simulink model "Trim_Model"  (R2014b)
settings: Solver=ode23tb  StartTime=0.0  StopTime=inf  FixedStep=0.001  MaxStep=0.01  RelTol=1e-5
values from neighbouring files (symbols this model uses):
  A_x = 0.015    [SetupComplete.m]
  A_y = A_x    (= 0.015)    [SetupComplete.m]
  A_z = 0.16    [SetupComplete.m]
  C_x = 1.2    [SetupComplete.m]
  C_y = C_x    (= 1.2)    [SetupComplete.m]
  C_z = 2.2    [SetupComplete.m]
  CG_0 = [0,0,0.02]'    [SetupComplete.m]
  h = 0.08    [SetupComplete.m]
  h_M = 0.064    [SetupComplete.m]
  I_BAC_0 = [ Ix,0,Ixz;0,Iy,0;Ixz,0,Iz]    [SetupComplete.m]
  l = 0.345    [SetupComplete.m]
  l_arm = 0.264    [SetupComplete.m]
  m = 3.51    [SetupComplete.m]
  m_0 = 2.61    [SetupComplete.m]
  m_M = 0.300    (= 0.3)    [SetupComplete.m]
  rho = 1.15    [SetupComplete.m]
  Rotation_sign = [ 1,-1,-1]    [SetupComplete.m]
undefined symbols (not defined in the file or in its folder): Throttle_Hover
libraries: simulink_extras x5, XXCopter_C x3, dspmtrx3 x2, aerolibtransform2 x1
settings Model: ExtModeTrigDuration=5000  Creator=DavidTorres  LastModifiedBy=david.torres
settings SolverCC: SolverResetMethod=Robust  PositivePriorityOrder=on
settings DataIOCC: ExternalInput=getinputstruct(op_trim1)  InitialState=getstatestruct(op_trim1)  SignalLoggingSaveFormat=ModelDataLogs  Refine=10
settings OptimizationCC: InlineParams=on  ExpressionDepthLimit=2147483647
settings DebuggingCC: UnderspecifiedInitializationDetection=Classic  MergeDetectMultiDrivingBlocksExec=none  FcnCallInpInsideContextMsg=UseLocalSettings  StateNameClashWarn=warning
settings RTWCC: SystemTargetFile=quarc_windows.tlc  TemplateMakefile=quarc_default_tmf  Description=QUARC Win32 Target  ProcessScript=quarc_windows_make_rtw_hook
settings STFCustomTargetCC: TargetPreCompLibLocation=C:\PROGRA~2\QUARC\lib\2011a\windows\release  CodeReplacementLibrary=C89/C90 (ANSI)  GeneratePreprocessorConditionals=Disable all  CPPClassGenCompliant=on  SystemTargetFile=quarc_windows.tlc
settings GRTTargetCC: TargetPreCompLibLocation=C:\PROGRA~2\QUARC\lib\2011a\windows\release  CodeReplacementLibrary=C89/C90 (ANSI)  ParMdlRefBuildCompliant=off  CompOptLevelCompliant=off  ConcurrentExecutionCompliant=off  CombineOutputUpdateFcns=off  MatFileLogging=off  GRTInterface=on  ExtMode=on  ExtModeMexFile=quarc_comm

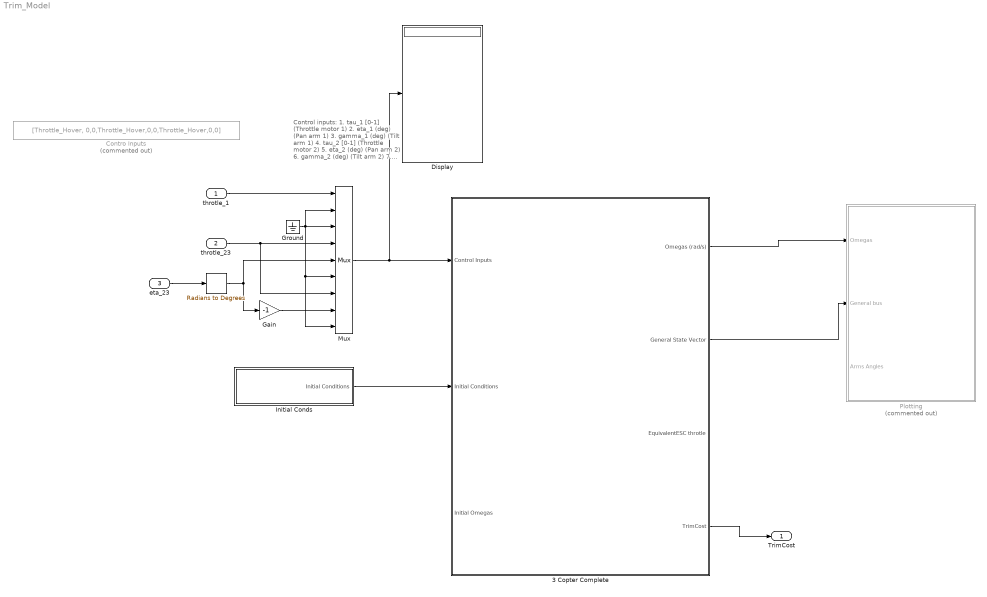
== system Trim_Model ==
  note: Control inputs:
      | 1. tau_1 [0-1] (Throttle motor 1)
      | 2. eta_1 (deg)  (Pan arm 1)
      | 3. gamma_1 (deg)  (Tilt arm 1)
      |
      | 4. tau_2 [0-1] (Throttle motor 2)
      | 5. eta_2 (deg)  (Pan arm 2)
      | 6. gamma_2 (deg)  (Tilt arm 2)
      |
      | 7. tau_3 [0-1] (Throttle motor 3)
      | 8. eta_3 (deg)  (Pan arm  3)
      | 9. gamma_3 (deg)  (Tilt arm 3)
  throtle_1 : Inport
  throtle_23 : Inport  Port=2
  eta_23 : Inport  Port=3
  " " : simulink_extras/Transformations/Radians to Degrees
  3 Copter Complete : Subsystem  TreatAsAtomicUnit=on
  Contro Inputs : Constant  Commented=on  Value=[Throttle_Hover, 0,0,Throttle_Hover,0,0,Throttle_Hover,0,0]
  Display : Display
  Gain : Gain  Gain=-1
  Ground : Ground
  Initial Conds : Subsystem  TreatAsAtomicUnit=on
  Mux : Mux  Inputs=9
  Plotting : Subsystem  Commented=on
  TrimCost : Outport
  wires:
  Initial Conds/1(Initial Conditions) -> 3 Copter Complete/2(Initial Conditions)
  Mux/1 -> Display/1, 3 Copter Complete/1(Control Inputs)
  3 Copter Complete/2(General State Vector) -> Plotting/2(General bus)
  3 Copter Complete/1(Omegas (rad/s)) -> Plotting/1(Omegas)
  ? -> Plotting/3(Arms Angles)
  3 Copter Complete/4(TrimCost) -> TrimCost/1
  throtle_1/1 -> Mux/1
  throtle_23/1 -> Mux/7, Mux/4
  Ground/1 -> Mux/2, Mux/6, Mux/9, Mux/3
  eta_23/1 -> " "/1
  " "/1 -> Gain/1, Mux/5
  Gain/1 -> Mux/8

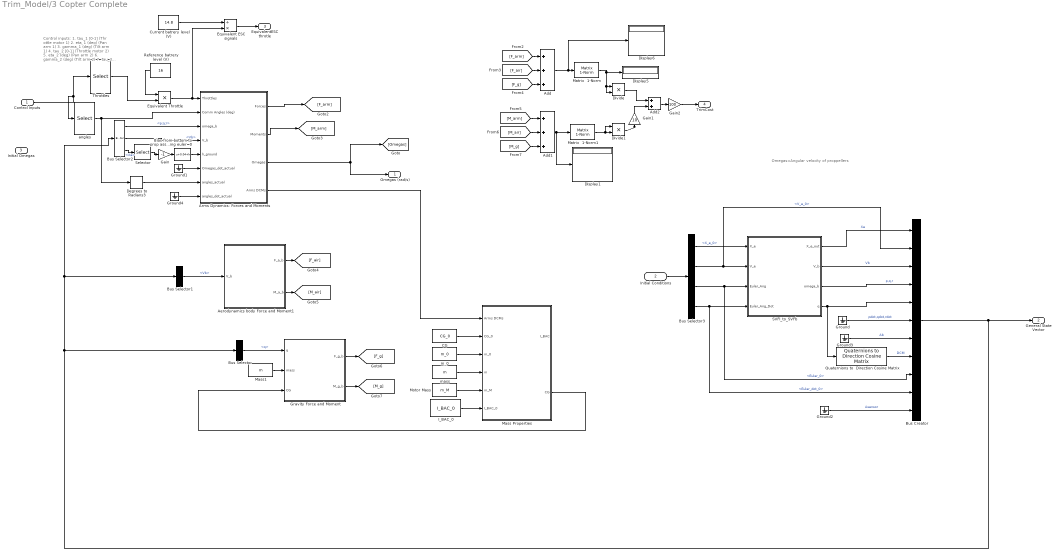
== system Trim_Model/3 Copter Complete ==
  note: Omegas=Angular velocity of proppellers
  note: Control inputs:
      | 1. tau_1 [0-1] (Thr ottle motor 1)
      | 2. eta_1 (deg)  (Pan arm 1)
      | 3. gamma_1 (deg)  (Tilt arm 1)
      |
      | 4. tau_2 [0-1] (Throttle motor 2)
      | 5. eta_2 (deg)  (Pan arm 2)
      | 6. gamma_2 (deg)  (Tilt arm 2)
      |
      | 7. tau_3 [0-1] (Throttle motor 3)
      | 8. eta_3 (deg)  (Pan arm  3)
      | 9. gamma_3 (deg)  (Tilt arm 3)
  Control Inputs : Inport
  Initial Conditions : Inport  Port=2
  Initial Omegas : Inport  Port=3
  Add : Sum  Inputs=+++
  Add1 : Sum  Inputs=+++
  Add2 : Sum
  Aerodynamics body Force and Moment1 : MATLAB Function  TreatAsAtomicUnit=on
  Arms Dynamics: Forces and Moments : Subsystem
  Bias from bottom to prop assuming euler=0 : Bias  Bias=0.04+h
  Bus Creator : BusCreator  Inputs=11
  Bus Selector : BusSelector  OutputSignals=q
  Bus Selector1 : BusSelector  OutputSignals=Vb
  Bus Selector2 : BusSelector  OutputSignals=p;q;r,Vb,Xe
  Bus Selector3 : BusSelector  OutputSignals=X_e_0,V_e_0,Euler_0,Euler_dot_0
  CG : Constant  Value=CG_0
  Current batrery level (V) : Constant  Value=14.8
  Degrees to Radians3 : simulink_extras/Transformations/Degrees to Radians
  Display1 : Display
  Display5 : Display
  Display6 : Display
  Divide : Product  Inputs=**
  Divide1 : Product  Inputs=**
  Equivalent ESC signals : Product  Inputs=/*
  Equivalent Throttle : Product  Inputs=**
  Gain : Gain  Gain=-1
  Gain1 : Gain  Gain=10
  Gain2 : Gain  Gain=100
  Gravity Force and Moment : MATLAB Function  TreatAsAtomicUnit=on
  Ground{,1..4} (5 alike) : Ground
  I_BAC_0 : Constant  Value=I_BAC_0
  Mass Properties : Subsystem  TreatAsAtomicUnit=on
  Mass1 : Constant  Value=m
  Matrix  1-Norm : dspmtrx3/Matrix  1-Norm  outputDataTypeStr=Inherit: Same as accumulator  outputLastDataTypeStr=Inherit: Same as accumulator  outputMin=[]  outputMax=[]  roundingMode=Floor  overflowMode=off
  Matrix  1-Norm1 : dspmtrx3/Matrix  1-Norm  outputDataTypeStr=Inherit: Same as accumulator  outputLastDataTypeStr=Inherit: Same as accumulator  outputMin=[]  outputMax=[]  roundingMode=Floor  overflowMode=off
  Motor Mass : Constant  Value=m_M
  Quaternions to  Direction Cosine Matrix : aerolibtransform2/Quaternions to  Direction Cosine Matrix
  Reference batrery level (V) : Constant  Value=16
  SVFI_to_SVFb : MATLAB Function  TreatAsAtomicUnit=on
  Selector : Selector  InputPortWidth=3  Indices=3
  Throttles : Selector  InputPortWidth=9  Indices=[1,4,7]
  "angles " : Selector  InputPortWidth=9  Indices=[2,3,5,6,8,9]
  m_0 : Constant  Value=m_0
  mass : Constant  Value=m
  Omegas (rad/s) : Outport
  General State Vector : Outport  Port=2
  EquivalentESC throtle : Outport  Port=3
  TrimCost : Outport  Port=4
  wires:
  SVFI_to_SVFb/3(omega_b) -> Bus Creator/4  "p,q,r"
  SVFI_to_SVFb/2(V_b) -> Bus Creator/3  "Vb"
  SVFI_to_SVFb/4(q) -> Quaternions to  Direction Cosine Matrix/1, Bus Creator/5
  Ground/1 -> Bus Creator/6  "pdot,qdot,rdot"
  SVFI_to_SVFb/1(X_e_out) -> Bus Creator/1  "Xe"
  Ground3/1 -> Bus Creator/7  "Ab"
  Bus Selector/1 -> Gravity Force and Moment/1(q)  "<q>"
  Bus Selector1/1 -> Aerodynamics body Force and Moment1/1(V_b)  "<Vb>"
  Bus Selector2/1 -> Arms Dynamics: Forces and Moments/3(omega_b)  "<p;q;r>"
  Bus Selector2/2 -> Arms Dynamics: Forces and Moments/4(V_b)  "<Vb>"
  Mass1/1 -> Gravity Force and Moment/2(mass)
  Mass Properties/2(CG) -> Gravity Force and Moment/3(CG)
  Bus Selector2/3 -> Selector/1  "<Xe>"
  Selector/1 -> Gain/1
  Arms Dynamics: Forces and Moments/1(Forces) -> [F_arm]
  Arms Dynamics: Forces and Moments/2(Moments) -> [M_arm]
  Aerodynamics body Force and Moment1/1(F_a_b) -> [F_air]
  Aerodynamics body Force and Moment1/2(M_a_b) -> [M_air]
  Gravity Force and Moment/1(F_g_b) -> [F_g]
  Gravity Force and Moment/2(M_g_b) -> [M_g]
  [F_arm] -> Add/1
  [F_air] -> Add/2
  [F_g] -> Add/3
  [M_arm] -> Add1/1
  [M_g] -> Add1/3
  [M_air] -> Add1/2
  Ground2/1 -> Bus Creator/11  "Asensor"
  Throttles/1 -> Equivalent Throttle/2
  Control Inputs/1 -> "angles "/1, Throttles/1
  "angles "/1 -> Arms Dynamics: Forces and Moments/2(Comm Angles (deg)), Degrees to Radians3/1
  Arms Dynamics: Forces and Moments/4(Arms DCMs) -> Mass Properties/1(Arms DCMs)
  CG/1 -> Mass Properties/2(CG_0)
  Motor Mass/1 -> Mass Properties/5(m_M)
  I_BAC_0/1 -> Mass Properties/6(I_BAC_0)
  m_0/1 -> Mass Properties/3(m_0)
  mass/1 -> Mass Properties/4(m)
  Arms Dynamics: Forces and Moments/3(Omegas) -> [Omegas], Omegas (rad/s)/1
  Bus Creator/1 -> Bus Selector2/1, Bus Selector1/1, Bus Selector/1, General State Vector/1
  Equivalent Throttle/1 -> Arms Dynamics: Forces and Moments/1(Throttles), Equivalent ESC signals/2
  Reference batrery level (V)/1 -> Equivalent Throttle/1
  Current batrery level (V)/1 -> Equivalent ESC signals/1
  Equivalent ESC signals/1 -> EquivalentESC throtle/1
  Initial Conditions/1 -> Bus Selector3/1
  Bus Selector3/1 -> SVFI_to_SVFb/1(X_e)  "<X_e_0>"
  Bus Selector3/2 -> Bus Creator/2, SVFI_to_SVFb/2(V_e)  "<V_e_0>"
  Bus Selector3/3 -> Bus Creator/9, SVFI_to_SVFb/3(Euler_Ang)  "<Euler_0>"
  Bus Selector3/4 -> Bus Creator/10, SVFI_to_SVFb/4(Euler_Ang_Dot)  "<Euler_dot_0>"
  Quaternions to  Direction Cosine Matrix/1 -> Bus Creator/8  "DCM"
  Add/1 -> Display6/1, Matrix  1-Norm/1
  Add1/1 -> Display1/1, Matrix  1-Norm1/1
  Add2/1 -> Gain2/1
  Gain1/1 -> Add2/2
  Matrix  1-Norm1/1 -> Divide1/1, Divide1/2
  Matrix  1-Norm/1 -> Divide/2, Divide/1, Display5/1
  Gain2/1 -> TrimCost/1
  Divide/1 -> Add2/1
  Divide1/1 -> Gain1/1
  Degrees to Radians3/1 -> Arms Dynamics: Forces and Moments/7(angles_actual)
  Ground1/1 -> Arms Dynamics: Forces and Moments/6(Omegas_dot_actual)
  Ground4/1 -> Arms Dynamics: Forces and Moments/8(angles_dot_actual)
  Gain/1 -> Bias from bottom to prop assuming euler=0/1
  Bias from bottom to prop assuming euler=0/1 -> Arms Dynamics: Forces and Moments/5(h_ground)

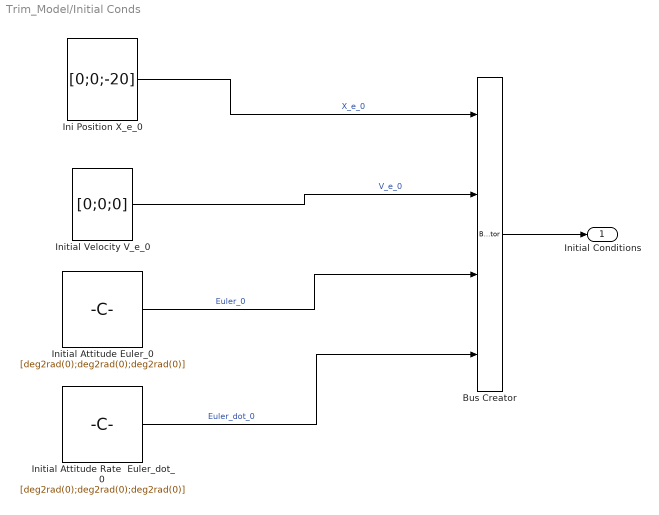
== system Trim_Model/Initial Conds ==
  Bus Creator : BusCreator
  Ini Position X_e_0 : Constant  Value=[0;0;-20]
  Initial Attitude Euler_0 : Constant  Value=[deg2rad(0);deg2rad(0);deg2rad(0)]
  Initial Attitude Rate  Euler_dot_0 : Constant  Value=[deg2rad(0);deg2rad(0);deg2rad(0)]
  Initial Velocity V_e_0 : Constant  Value=[0;0;0]
  Initial Conditions : Outport
  wires:
  Ini Position X_e_0/1 -> Bus Creator/1  "X_e_0"
  Initial Velocity V_e_0/1 -> Bus Creator/2  "V_e_0"
  Initial Attitude Euler_0/1 -> Bus Creator/3  "Euler_0"
  Initial Attitude Rate  Euler_dot_0/1 -> Bus Creator/4  "Euler_dot_0"
  Bus Creator/1 -> Initial Conditions/1

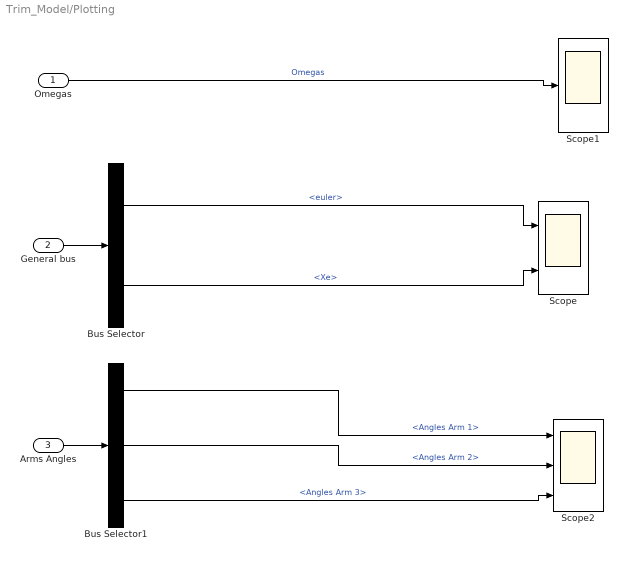
== system Trim_Model/Plotting ==
  Omegas : Inport
  General bus : Inport  Port=2
  Arms Angles : Inport  Port=3
  Bus Selector : BusSelector  OutputSignals=euler,Xe
  Bus Selector1 : BusSelector  OutputSignals=Angles Arm 1,Angles Arm 2,Angles Arm 3
  Scope : Scope  NumInputPorts=2
      settings: YMin=-3.5~-110  YMax=3.5~40
  Scope1 : Scope
      settings: TimeRange=5  YMin=0  YMax=700
  Scope2 : Scope  NumInputPorts=3
      settings: ShowLegends=on  YMin=-5~-5~-5  YMax=5~5~5  SaveName=ScopeData2
  wires:
  General bus/1 -> Bus Selector/1
  Bus Selector/1 -> Scope/1  "<euler>"
  Omegas/1 -> Scope1/1  "Omegas"
  Arms Angles/1 -> Bus Selector1/1
  Bus Selector1/3 -> Scope2/3  "<Angles Arm 3>"
  Bus Selector1/2 -> Scope2/2  "<Angles Arm 2>"
  Bus Selector1/1 -> Scope2/1  "<Angles Arm 1>"
  Bus Selector/2 -> Scope/2  "<Xe>"

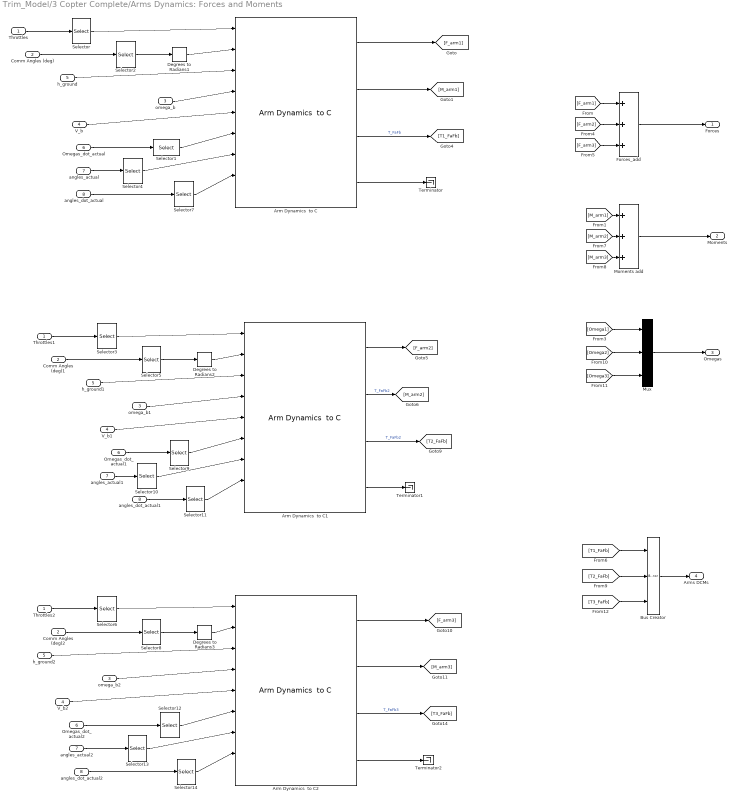
== system Trim_Model/3 Copter Complete/Arms Dynamics: Forces and Moments ==
  Throttles : Inport
  Comm Angles (deg) : Inport  Port=2
  omega_b : Inport  Port=3
  V_b : Inport  Port=4
  h_ground : Inport  Port=5
  Omegas_dot_actual : Inport  Port=6
  angles_actual : Inport  Port=7
  angles_dot_actual : Inport  Port=8
  Arm Dynamics  to C : XXCopter_C/Arm Dynamics  to C  Rot_sign=Rotation_sign(1)  arm_hub_pos=l*[1;0;0]  Arm_axis=[l_arm;0;0]  arm_num=1  eta_dir=[1;0;0]  gamma_dir=[0;1;0]  J_T=J_T  J_FA=J_FA  h=h  switch_val=direct_feedforward  omega_n=40  xi=0.8  eta_inf_lim=deg2rad(-180)  eta_sup_lim=deg2rad(180)  gamma_inf_lim=deg2rad(-90)  gamma_sup_lim=deg2rad(30)
      link override ESC+Motor Dynamcis  to C/2-D Torque-Throttle-Omega Map: BreakpointsForDimension1=TO_map_Throtle  BreakpointsForDimension2=Throtle_TTO_vec
  Arm Dynamics  to C1 : XXCopter_C/Arm Dynamics  to C  Rot_sign=Rotation_sign(2)  arm_hub_pos=l*[-1/2;sqrt(3)/2;0]  Arm_axis=[0;l_arm;0]  arm_num=2  eta_dir=[0;1;0]  gamma_dir=[1;0;0]  J_T=J_T  J_FA=J_FA  h=h  switch_val=direct_feedforward  omega_n=40  xi=0.8  eta_inf_lim=deg2rad(-180)  eta_sup_lim=deg2rad(180)  gamma_inf_lim=deg2rad(-30)  gamma_sup_lim=deg2rad(90)
  Arm Dynamics  to C2 : XXCopter_C/Arm Dynamics  to C  Rot_sign=Rotation_sign(3)  arm_hub_pos=l*[-1/2;-sqrt(3)/2;0]  Arm_axis=[0;-l_arm;0]  arm_num=3  eta_dir=[0;1;0]  gamma_dir=[1;0;0]  J_T=J_T  J_FA=J_FA  h=h  switch_val=direct_feedforward  omega_n=40  xi=0.8  eta_inf_lim=deg2rad(-180)  eta_sup_lim=deg2rad(180)  gamma_inf_lim=deg2rad(-90)  gamma_sup_lim=deg2rad(30)
  Bus Creator : BusCreator  Inputs=3
  Comm Angles (deg)1 : InportShadow  Port=2
  Comm Angles (deg)2 : InportShadow  Port=2
  Degrees to Radians1 : simulink_extras/Transformations/Degrees to Radians
  Degrees to Radians2 : simulink_extras/Transformations/Degrees to Radians
  Degrees to Radians3 : simulink_extras/Transformations/Degrees to Radians
  Forces_add : Sum  Inputs=+++
  Moments add : Sum  Inputs=+++
  Mux : Mux  Inputs=3
  Omegas_dot_actual1 : InportShadow  Port=6
  Omegas_dot_actual2 : InportShadow  Port=6
  Selector : Selector  IndexMode=Zero-based  InputPortWidth=3  Indices=0
  Selector1 : Selector  IndexMode=Zero-based  InputPortWidth=3  Indices=0
  Selector10 : Selector  IndexMode=Zero-based  InputPortWidth=6  Indices=[2,3]
  Selector11 : Selector  IndexMode=Zero-based  InputPortWidth=6  Indices=[2,3]
  Selector12 : Selector  IndexMode=Zero-based  InputPortWidth=3  Indices=2
  Selector13 : Selector  IndexMode=Zero-based  InputPortWidth=6  Indices=[4,5]
  Selector14 : Selector  IndexMode=Zero-based  InputPortWidth=6  Indices=[4,5]
  Selector2 : Selector  IndexMode=Zero-based  InputPortWidth=6  Indices=[0,1]
  Selector3 : Selector  IndexMode=Zero-based  InputPortWidth=3
  Selector4 : Selector  IndexMode=Zero-based  InputPortWidth=6  Indices=[0,1]
  Selector5 : Selector  IndexMode=Zero-based  InputPortWidth=6  Indices=[2,3]
  Selector6 : Selector  IndexMode=Zero-based  InputPortWidth=3  Indices=2
  Selector7 : Selector  IndexMode=Zero-based  InputPortWidth=6  Indices=[0,1]
  Selector8 : Selector  IndexMode=Zero-based  InputPortWidth=6  Indices=[4,5]
  Selector9 : Selector  IndexMode=Zero-based  InputPortWidth=3
  Terminator : Terminator
  Terminator1 : Terminator
  Terminator2 : Terminator
  Throttles1 : InportShadow
  Throttles2 : InportShadow
  V_b1 : InportShadow  Port=4
  V_b2 : InportShadow  Port=4
  angles_actual1 : InportShadow  Port=7
  angles_actual2 : InportShadow  Port=7
  angles_dot_actual1 : InportShadow  Port=8
  angles_dot_actual2 : InportShadow  Port=8
  h_ground1 : InportShadow  Port=5
  h_ground2 : InportShadow  Port=5
  omega_b1 : InportShadow  Port=3
  omega_b2 : InportShadow  Port=3
  Forces : Outport
  Moments : Outport  Port=2
  Omegas : Outport  Port=3
  Arms DCMs : Outport  Port=4
  wires:
  Forces_add/1 -> Forces/1
  Moments add/1 -> Moments/1
  Mux/1 -> Omegas/1
  [F_arm1] -> Forces_add/1
  [M_arm1] -> Moments add/1
  [Omega1] -> Mux/1
  [F_arm2] -> Forces_add/2
  [F_arm3] -> Forces_add/3
  [Omega2] -> Mux/2
  [Omega3] -> Mux/3
  [M_arm3] -> Moments add/3
  [M_arm2] -> Moments add/2
  Bus Creator/1 -> Arms DCMs/1
  [T1_FaFb] -> Bus Creator/1
  [T2_FaFb] -> Bus Creator/2
  [T3_FaFb] -> Bus Creator/3
  Throttles/1 -> Selector/1
  Selector/1 -> Arm Dynamics  to C/1
  V_b/1 -> Arm Dynamics  to C/5
  h_ground/1 -> Arm Dynamics  to C/3
  Arm Dynamics  to C/1 -> [F_arm1]
  Arm Dynamics  to C/2 -> [M_arm1]
  omega_b/1 -> Arm Dynamics  to C/4
  Degrees to Radians1/1 -> Arm Dynamics  to C/2
  Comm Angles (deg)/1 -> Selector2/1
  Selector2/1 -> Degrees to Radians1/1
  Arm Dynamics  to C/3 -> [T1_FaFb]  "T_FaFb"
  Throttles1/1 -> Selector3/1
  Selector3/1 -> Arm Dynamics  to C1/1
  V_b1/1 -> Arm Dynamics  to C1/5
  h_ground1/1 -> Arm Dynamics  to C1/3
  omega_b1/1 -> Arm Dynamics  to C1/4
  Degrees to Radians2/1 -> Arm Dynamics  to C1/2
  Comm Angles (deg)1/1 -> Selector5/1
  Selector5/1 -> Degrees to Radians2/1
  Arm Dynamics  to C1/3 -> [T2_FaFb]  "T_FaFb2"
  Throttles2/1 -> Selector6/1
  Selector6/1 -> Arm Dynamics  to C2/1
  V_b2/1 -> Arm Dynamics  to C2/5
  h_ground2/1 -> Arm Dynamics  to C2/3
  Arm Dynamics  to C2/1 -> [F_arm3]
  Arm Dynamics  to C2/2 -> [M_arm3]
  omega_b2/1 -> Arm Dynamics  to C2/4
  Degrees to Radians3/1 -> Arm Dynamics  to C2/2
  Comm Angles (deg)2/1 -> Selector8/1
  Selector8/1 -> Degrees to Radians3/1
  Arm Dynamics  to C2/3 -> [T3_FaFb]  "T_FaFb3"
  Arm Dynamics  to C/4 -> Terminator/1
  Arm Dynamics  to C1/4 -> Terminator1/1
  Arm Dynamics  to C2/4 -> Terminator2/1
  Arm Dynamics  to C1/1 -> [F_arm2]
  Arm Dynamics  to C1/2 -> [M_arm2]  "T_FaFb2"
  Omegas_dot_actual/1 -> Selector1/1
  Selector1/1 -> Arm Dynamics  to C/6
  angles_actual/1 -> Selector4/1
  Selector4/1 -> Arm Dynamics  to C/7
  angles_dot_actual/1 -> Selector7/1
  Selector7/1 -> Arm Dynamics  to C/8
  Omegas_dot_actual1/1 -> Selector9/1
  Selector9/1 -> Arm Dynamics  to C1/6
  Selector10/1 -> Arm Dynamics  to C1/7
  angles_dot_actual1/1 -> Selector11/1
  angles_actual1/1 -> Selector10/1
  Selector11/1 -> Arm Dynamics  to C1/8
  Omegas_dot_actual2/1 -> Selector12/1
  Selector12/1 -> Arm Dynamics  to C2/6
  Selector13/1 -> Arm Dynamics  to C2/7
  angles_dot_actual2/1 -> Selector14/1
  angles_actual2/1 -> Selector13/1
  Selector14/1 -> Arm Dynamics  to C2/8

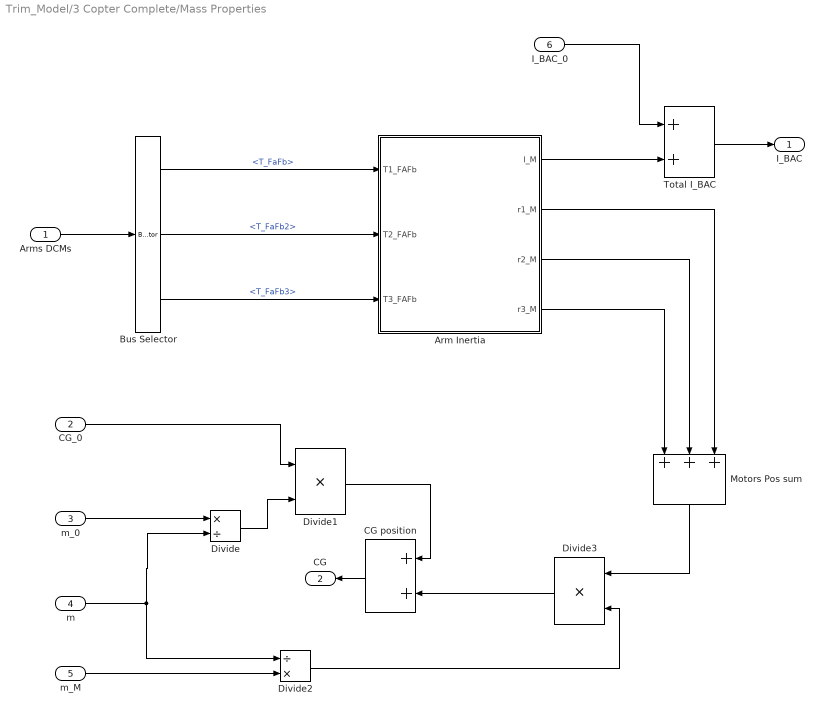
== system Trim_Model/3 Copter Complete/Mass Properties ==
  Arms DCMs : Inport
  CG_0 : Inport  Port=2
  m_0 : Inport  Port=3
  m : Inport  Port=4
  m_M : Inport  Port=5
  I_BAC_0 : Inport  Port=6
  Arm Inertia : MATLAB Function  TreatAsAtomicUnit=on
  Bus Selector : BusSelector  OutputSignals=T_FaFb,T_FaFb2,T_FaFb3
  CG position : Sum
  Divide : Product  Inputs=*/
  Divide1 : Product  Inputs=**
  Divide2 : Product  Inputs=/*
  Divide3 : Product  Inputs=**
  Motors Pos sum : Sum  Inputs=+++
  Total I_BAC : Sum
  I_BAC : Outport
  CG : Outport  Port=2
  wires:
  Arms DCMs/1 -> Bus Selector/1
  Bus Selector/3 -> Arm Inertia/3(T3_FAFb)  "<T_FaFb3>"
  Bus Selector/2 -> Arm Inertia/2(T2_FAFb)  "<T_FaFb2>"
  Bus Selector/1 -> Arm Inertia/1(T1_FAFb)  "<T_FaFb>"
  Total I_BAC/1 -> I_BAC/1
  m_0/1 -> Divide/1
  m/1 -> Divide/2, Divide2/1
  CG_0/1 -> Divide1/1
  Divide/1 -> Divide1/2
  m_M/1 -> Divide2/2
  CG position/1 -> CG/1
  Divide1/1 -> CG position/1
  Motors Pos sum/1 -> Divide3/1
  Divide2/1 -> Divide3/2
  Divide3/1 -> CG position/2
  Arm Inertia/3(r2_M) -> Motors Pos sum/2
  Arm Inertia/4(r3_M) -> Motors Pos sum/1
  Arm Inertia/1(I_M) -> Total I_BAC/2
  I_BAC_0/1 -> Total I_BAC/1
  Arm Inertia/2(r1_M) -> Motors Pos sum/3

== matlab function Trim_Model/3 Copter Complete/Gravity Force and Moment ==
  data: q input; F_g_b output; M_g_b output; mass input; CG input; g parameter
function [F_g_b,M_g_b]   = Grav_Forces_and_Mom( q,mass,CG, g)

Prod=HamiltonProduct([q(1);-q(2);-q(3);-q(4)],HamiltonProduct([0;0;0;mass*g],[q(1);q(2);q(3);q(4)]) ); % q* . g .q

F_g_b= Prod(2:4);
M_g_b=cross(CG,F_g_b);
end

== matlab function Trim_Model/3 Copter Complete/Aerodynamics body Force and Moment1 ==
  data: V_b input; F_a_b output; M_a_b output; rho parameter; C_x parameter; C_y parameter; C_z parameter; A_x parameter; A_y parameter; A_z parameter
function [F_a_b,M_a_b]   = Aero_body_Forces_and_Mom( V_b, rho,C_x,C_y,C_z,A_x,A_y,A_z)


F_a_b=1/2*rho*(V_b*V_b')*[C_x*A_x;C_y*A_y;C_z*A_z].*( - V_b./(norm(V_b)+eps) );
M_a_b=[0;0;0];
end

== matlab function Trim_Model/3 Copter Complete/Mass Properties/Arm Inertia ==
  data: T1_FAFb input; T2_FAFb input; T3_FAFb input; I_M output; l parameter; h_M parameter; m_M parameter; r1_M output; r2_M output; r3_M output
function [I_M,r1_M,r2_M,r3_M]  = Arm1_inertia(T1_FAFb,T2_FAFb,T3_FAFb, l, h_M, m_M)


r1_M=[l;0;0]+T1_FAFb*[0;0;-h_M];
r2_M=[-1/2*l;sqrt(3)/2*l;0]+T2_FAFb*[0;0;-h_M];
r3_M=[-1/2*l;-sqrt(3)/2*l;0]+T3_FAFb*[0;0;-h_M];


I_M1 = m_M*[ r1_M(2)^2+r1_M(3)^2,r1_M(1)*r1_M(2),r1_M(1)*r1_M(3);...
            r1_M(1)*r1_M(2), r1_M(1)^2+r1_M(3)^2, r1_M(2)*r1_M(3);...
            r1_M(1)*r1_M(3),r1_M(2)*r1_M(3), r1_M(1)^2+r1_M(2)^2];
I_M2 = m_M*[ r2_M(2)^2+r2_M(3)^2,r2_M(1)*r2_M(2),r2_M(1)*r2_M(3);...
            r2_M(1)*r2_M(2), r2_M(1)^2+r2_M(3)^2, r2_M(2)*r2_M(3);...
            r2_M(1)*r2_M(3),r2_M(2)*r2_M(3), r2_M(1)^2+r2_M(2)^2];
I_M3 = m_M*[ r3_M(2)^2+r3_M(3)^2,r3_M(1)*r3_M(2),r3_M(1)*r3_M(3);...
            r3_M(1)*r3_M(2), r3_M(1)^2+r3_M(3)^2, r3_M(2)*r3_M(3);...
            r3_M(1)*r3_M(3),r3_M(2)*r3_M(3), r3_M(1)^2+r3_M(2)^2];

I_M = I_M1+I_M2+I_M3;

== matlab function Trim_Model/3 Copter Complete/SVFI_to_SVFb ==
  data: X_e input; V_e input; X_e_out output; V_b output; omega_b output; Euler_Ang input; Euler_Ang_Dot input; q output
function [X_e_out,V_b, omega_b ,q]=SVFI_to_SVFb(X_e,V_e, Euler_Ang,Euler_Ang_Dot)

xp=V_e(1);
yp=V_e(2);
zp=V_e(3);

phi=Euler_Ang(1);
theta=Euler_Ang(2);
psi=Euler_Ang(3);
phip=Euler_Ang_Dot(1);
thetap=Euler_Ang_Dot(2);
psip=Euler_Ang_Dot(3);

%%
X_e_out=X_e;

q = QuaternionfromEuler(phi,theta,psi); 



HamOut=HamiltonProduct([q(1);-q(2);-q(3);-q(4)],HamiltonProduct([0;xp;yp;zp],[q(1);q(2);q(3);q(4)]) );% q* . v . q
V_b=HamOut(2:4);

omega_b=[phip-psip*sin(theta)  ;
         thetap*cos(phi)+psip*cos(theta)*sin(phi);
            -thetap*sin(phi)+psip*cos(theta)*cos(phi)  ];% Ya que es solo una operacion aislada utilizaremos la ecuaciones con rel trigonometricas
end
function [q]=QuaternionfromEuler(phi,theta,psi)
% options=optimset('MaxFunEvals',3000);
% q=fsolve(@QUATERNIONEULER,[0.6,0.4,0.5,0.4]); % Hay que acertar con los angulos poniendo diferentes valores iniciales del quaternion
%     function F=QUATERNIONEULER(q)
%         F=[ tan(phi)-(2*q(3)*q(4)-2*q(1)*q(2))/(2*q(1)^2+2*q(4)^2-1)  ;
%             sin(-theta)-2*q(2)*q(4)-2*q(1)*q(3);
%             tan(psi)-(2*q(2)*q(3)-2*q(1)*q(4))/(2*q(1)^2+2*q(2)^2-1);
%             q(1)^2+q(2)^2+q(3)^2+q(4)^2-1];
%     end  % Este algoritmo da q* !!!!!

q=[ cos(psi/2)*cos(theta/2)*cos(phi/2)+ sin(psi/2)*sin(theta/2)*sin(phi/2) ;
      cos(psi/2)*cos(theta/2)*sin(phi/2)- sin(psi/2)*sin(theta/2)*cos(phi/2) ;
       cos(psi/2)*sin(theta/2)*cos(phi/2)+ sin(psi/2)*cos(theta/2)*sin(phi/2)   ;
        sin(psi/2)*cos(theta/2)*cos(phi/2)- cos(psi/2)*sin(theta/2)*sin(phi/2)      ]; % Esto nos da q !!!
end
